simulink model "MagLev"  (R2015a)
settings: Solver=ode5  SolverMode=SingleTasking  StartTime=0.0  StopTime=5  FixedStep=1e-3  MaxStep=0.001  RelTol=1e-3  AbsTol=1e-5
PreLoadFcn:
  | Ts=1e-3;
libraries: vrlib x3
Description:
  | Magnetic Levitation Model
  | 
  | vrmaglev is an example showing the interaction between dynamic models in Simulink(R)
  | and virtual worlds. The Simulink model represents the HUMUSOFT(R) CE152 Magnetic Levitation
  | educational / presentation scale model. (http://www.humusoft.com/link/models)
  | 
  | The plant model is controlled by a PID controller with feed forward to cope with the nonlinearity
  | of the magnetic levitation system.
  | 
  | The position of the ball responds to the changing value of the setpoint. You can observe
  | this change not only in the Scope window, but also in a viewer window displaying
  | the virtual world. Note that the position of the ball represents the real dynamics of the system.
  | If you switch the VRML viewer to the Camera 3 viewpoint, you can observe and control the ball easier.
  | 
  | There are two possible methods of setting the ball position setpoint - using a Signal Generator
  | and visually by clicking at a desired position in the virtual reality scene.
  | 
  | In the virtual scene, a VRML sensor is defined. If you click in the space between the magnetic coil
  | and the bottom plate, VRML sensor is updated and its value is read into Simulink model using the
  | VR Source block.
settings Model: FPTRunName=Active  CovMetricSettings=d  CovSFcnEnable=off  ExtModeTrigDuration=5000  ExtModeTrigLevel=0.500000  Creator=The MathWorks Inc.  LastModifiedBy=Logan
settings DataIOCC: LimitDataPoints=off  SaveOutput=off  SaveTime=off  SignalLoggingName=logsOut
settings OptimizationCC: BlockReduction=off  BooleanDataType=off  OptimizeBlockIOStorage=off  BufferReuse=off  GlobalBufferReuse=off  ExpressionFolding=off  ExpressionDepthLimit=2147483647  LocalBlockOutputs=off  InitFltsAndDblsToZero=on
settings DebuggingCC: UnderspecifiedInitializationDetection=Classic  MergeDetectMultiDrivingBlocksExec=none  CheckExecutionContextPreStartOutputMsg=on  CheckExecutionContextRuntimeOutputMsg=on  SignalResolutionControl=TryResolveAllWithWarning  MultiTaskDSMMsg=warning  MultiTaskCondExecSysMsg=none  FcnCallInpInsideContextMsg=UseLocalSettings  StateNameClashWarn=warning
settings HardwareCC: TargetUnknown=on
settings ModelReferenceCC: UpdateModelReferenceTargets=IfOutOfDate
settings RTWCC: RetainRTWFile=on
settings GRTTargetCC: TargetFcnLib=ansi_tfl_tmw.mat  CombineOutputUpdateFcns=off  GRTInterface=on

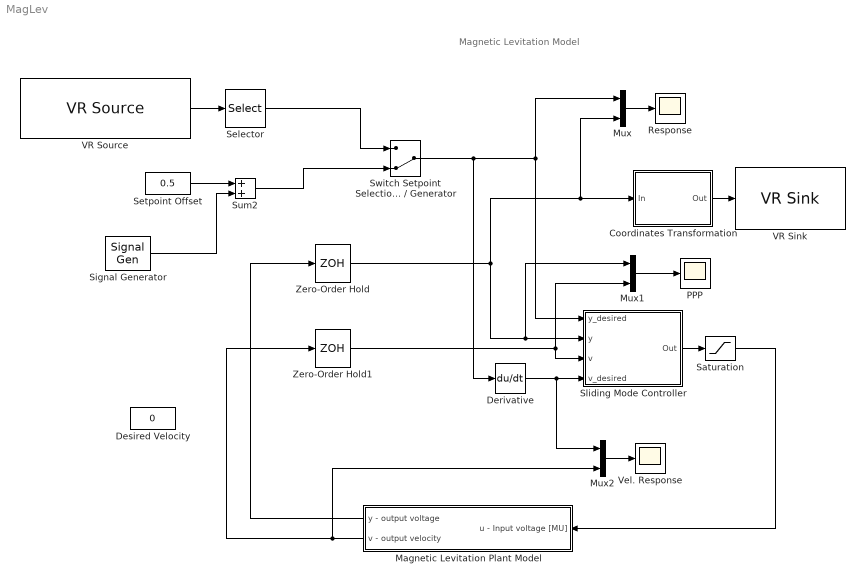
== system MagLev ==
  note: Magnetic Levitation Model
  Coordinates Transformation : Subsystem
  Derivative : Derivative
  Desired Velocity : Constant  Value=0
  Magnetic Levitation Plant Model : Subsystem
  Mux : Mux  Inputs=2
  Mux1 : Mux  Inputs=2
  Mux2 : Mux  Inputs=2
  PPP : Scope
      settings: TimeRange=5  YMin=0  YMax=1  SaveName=PhasePlane  MaxDataPoints=250  SampleInput=on  SampleTime=0.02
  Response : Scope
      settings: TimeRange=5  YMin=-0.0227122  YMax=1.027  SaveName=ResponseSMC  MaxDataPoints=250  SampleInput=on  SampleTime=0.02
  Saturation : Saturate  UpperLimit=1  LowerLimit=0  ZeroCross=off
  Selector : Selector  InputPortWidth=3  Indices=[2]
  Setpoint Offset : Constant  Value=0.5
  Signal Generator : SignalGenerator  Amplitude=0.25  Frequency=2  Units=rad/sec
  Sliding Mode Controller : Subsystem
  Sum2 : Sum  SaturateOnIntegerOverflow=on  InputSameDT=on  OutDataTypeStr=Inherit: Same as first input
  Switch Setpoint Selection Method Virtual Reality / Generator : ManualSwitch  CurrentSetting=0
  VR Sink : vrlib/VR Sink  InstantiateOnLoad=on  SampleTime=0.02  ViewEnable=on  RemoteChange=off  RemoteView=off  FieldsWritten=Ball.translation.3.1.1.double  WorldFileName=maglev.wrl  WorldDescription=VR Magnetic Levitation Model  AutoView=on  VideoDimensions=[]  AllowVariableSize=off
  VR Source : vrlib/VR Source  InstantiateOnLoad=on  SampleTime=0.1  ViewEnable=on  RemoteChange=off  RemoteView=off  FieldsRead=Grab_Sensor.translation_changed.3.1.1.double  WorldFileName=maglev.wrl  WorldDescription=VR Magnetic Levitation Model  AutoView=off  VideoDimensions=[]  AllowVariableSize=off
  Vel. Response : Scope
      settings: TimeRange=5  YMin=-0.0227122  YMax=1.027  DataFormat=Structure  MaxDataPoints=250  SampleInput=on  SampleTime=0.02
  Zero-Order Hold : ZeroOrderHold  SampleTime=Ts
  Zero-Order Hold1 : ZeroOrderHold  SampleTime=Ts
  wires:
  Zero-Order Hold/1 -> Coordinates Transformation/1(In), Mux/2, Mux1/1, Sliding Mode Controller/2(y)
  Switch Setpoint Selection Method Virtual Reality / Generator/1 -> Derivative/1, Sliding Mode Controller/1(y_desired), Mux/1
  Mux/1 -> Response/1
  Magnetic Levitation Plant Model/1(y - output voltage) -> Zero-Order Hold/1
  Coordinates Transformation/1(Out) -> VR Sink/1
  Saturation/1 -> Magnetic Levitation Plant Model/1(u - Input voltage [MU])
  Selector/1 -> Switch Setpoint Selection Method Virtual Reality / Generator/1
  VR Source/1 -> Selector/1
  Sliding Mode Controller/1(Out) -> Saturation/1
  Magnetic Levitation Plant Model/2(v - output velocity) -> Mux2/2, Zero-Order Hold1/1
  Zero-Order Hold1/1 -> Sliding Mode Controller/3(v), Mux1/2
  Mux1/1 -> PPP/1
  Signal Generator/1 -> Sum2/2
  Setpoint Offset/1 -> Sum2/1
  Sum2/1 -> Switch Setpoint Selection Method Virtual Reality / Generator/2
  Mux2/1 -> Vel. Response/1
  Derivative/1 -> Mux2/1, Sliding Mode Controller/4(v_desired)

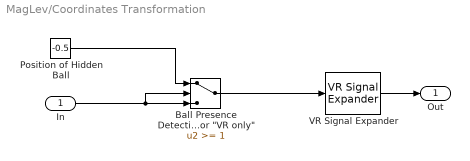
== system MagLev/Coordinates Transformation ==
  In : Inport
  "Ball Presence Detection Value > Threshold = Ball Not Present 1 for \"VR only\"" : Switch  Threshold=1  InputSameDT=on
  Position of Hidden Ball : Constant  Value=-0.5
  VR Signal Expander : vrlib/VR Signal Expander  outwidth=3  outidx=[2]
  Out : Outport
  wires:
  Position of Hidden Ball/1 -> "Ball Presence Detection Value > Threshold = Ball Not Present 1 for \"VR only\""/1
  In/1 -> "Ball Presence Detection Value > Threshold = Ball Not Present 1 for \"VR only\""/3, "Ball Presence Detection Value > Threshold = Ball Not Present 1 for \"VR only\""/2
  "Ball Presence Detection Value > Threshold = Ball Not Present 1 for \"VR only\""/1 -> VR Signal Expander/1
  VR Signal Expander/1 -> Out/1

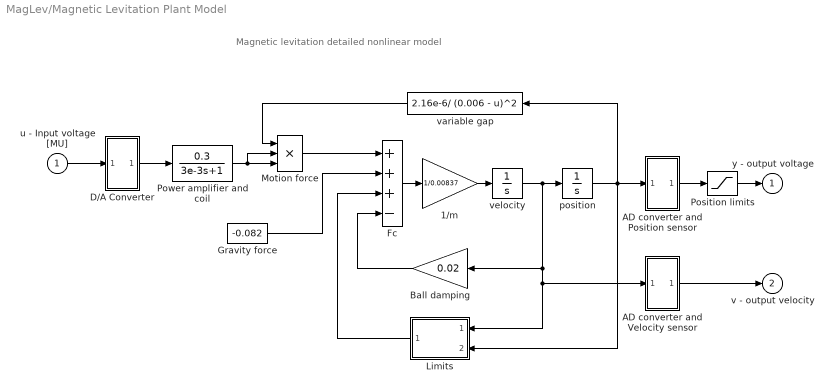
== system MagLev/Magnetic Levitation Plant Model ==
  note: Magnetic levitation
      | detailed nonlinear model
  u - Input voltage [MU] : Inport
  1/m : Gain  Gain=1/0.00837  SaturateOnIntegerOverflow=on  OutDataTypeStr=Inherit: Same as input  ParamDataTypeStr=Inherit: Same as input
  AD converter and Position sensor : Subsystem
      mask Display: disp('A/D')
  AD converter and Velocity sensor : Subsystem
      mask Display: disp('A/D')
  Ball damping : Gain  Gain=0.02  SaturateOnIntegerOverflow=on  OutDataTypeStr=Inherit: Same as input  ParamDataTypeStr=Inherit: Same as input
  D/A Converter : Subsystem
      mask Display: disp('D/A')
  Fc : Sum  Inputs=+++-  SaturateOnIntegerOverflow=on  InputSameDT=on  OutDataTypeStr=Inherit: Same as first input
  Gravity force : Constant  Value=-0.082
  Limits : Subsystem
      mask Display: disp('LIMIT')
  Motion force : Product  Inputs=3  SaturateOnIntegerOverflow=on  InputSameDT=on  OutDataTypeStr=Inherit: Same as first input
  Position limits : Saturate  UpperLimit=0.998  LowerLimit=0  ZeroCross=off
  Power amplifier and coil : TransferFcn  Numerator=[0.3]  Denominator=[3e-3 1]
  position : Integrator  LimitOutput=on  UpperSaturationLimit=0.005  LowerSaturationLimit=0  ZeroCross=off
  variable gap : Fcn  Expr=2.16e-6/ (0.006 - u)^2
  velocity : Integrator  UpperSaturationLimit=Inf  LowerSaturationLimit=-Inf  ZeroCross=off
  y - output voltage : Outport
  v - output velocity : Outport  Port=2
  wires:
  Ball damping/1 -> Fc/4
  variable gap/1 -> Motion force/1
  1/m/1 -> velocity/1
  Fc/1 -> 1/m/1
  Motion force/1 -> Fc/1
  Gravity force/1 -> Fc/2
  D/A Converter/1(out_1) -> Power amplifier and coil/1
  u - Input voltage [MU]/1 -> D/A Converter/1(in_1)
  AD converter and Position sensor/1(out_1) -> Position limits/1
  position/1 -> Limits/2(position), variable gap/1, AD converter and Position sensor/1(in_1)
  Limits/1(force) -> Fc/3
  Power amplifier and coil/1 -> Motion force/3, Motion force/2
  Position limits/1 -> y - output voltage/1
  AD converter and Velocity sensor/1(out_1) -> v - output velocity/1
  velocity/1 -> AD converter and Velocity sensor/1(in_1), Limits/1(velocity), Ball damping/1, position/1

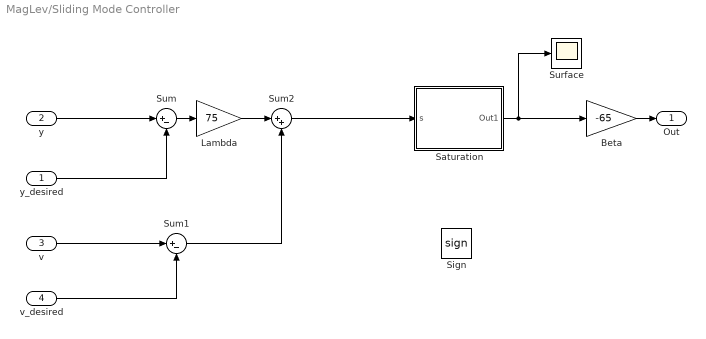
== system MagLev/Sliding Mode Controller ==
  y_desired : Inport
  y : Inport  Port=2
  v : Inport  Port=3
  v_desired : Inport  Port=4
  Beta : Gain  Gain=-65
  Lambda : Gain  Gain=75
  Saturation : Subsystem
  Sign : Signum
  Sum : Sum  Inputs=|+-
  Sum1 : Sum  Inputs=|+-
  Sum2 : Sum  Inputs=|++
  Surface : Scope
      settings: TimeRange=5  YMin=-3.15  YMax=-2.85  SaveName=ScopeData2  DataFormat=Structure  MaxDataPoints=250  SampleInput=on  SampleTime=0.02
  Out : Outport
  wires:
  v/1 -> Sum1/1
  v_desired/1 -> Sum1/2
  y/1 -> Sum/1
  y_desired/1 -> Sum/2
  Sum/1 -> Lambda/1
  Lambda/1 -> Sum2/1
  Sum1/1 -> Sum2/2
  Beta/1 -> Out/1
  Saturation/1(Out1) -> Surface/1, Beta/1
  Sum2/1 -> Saturation/1(s)

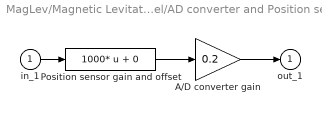
== system MagLev/Magnetic Levitation Plant Model/AD converter and Position sensor ==
  in_1 : Inport
  A/D converter gain : Gain  Gain=0.2  SaturateOnIntegerOverflow=on  OutDataTypeStr=Inherit: Same as input  ParamDataTypeStr=Inherit: Same as input
  Position sensor gain and offset : Fcn  Expr=1000* u + 0
  out_1 : Outport
  wires:
  in_1/1 -> Position sensor gain and offset/1
  Position sensor gain and offset/1 -> A/D converter gain/1
  A/D converter gain/1 -> out_1/1

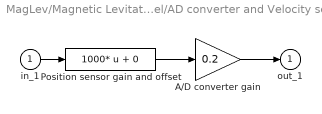
== system MagLev/Magnetic Levitation Plant Model/AD converter and Velocity sensor ==
  in_1 : Inport
  A/D converter gain : Gain  Gain=0.2  SaturateOnIntegerOverflow=on  OutDataTypeStr=Inherit: Same as input  ParamDataTypeStr=Inherit: Same as input
  Position sensor gain and offset : Fcn  Expr=1000* u + 0
  out_1 : Outport
  wires:
  in_1/1 -> Position sensor gain and offset/1
  Position sensor gain and offset/1 -> A/D converter gain/1
  A/D converter gain/1 -> out_1/1

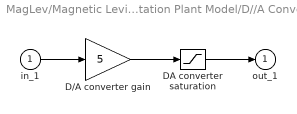
== system MagLev/Magnetic Levitation Plant Model/D//A Converter ==
  in_1 : Inport
  D/A converter gain : Gain  Gain=5  SaturateOnIntegerOverflow=on  OutDataTypeStr=Inherit: Same as input  ParamDataTypeStr=Inherit: Same as input
  DA converter saturation : Saturate  UpperLimit=5  LowerLimit=-5  ZeroCross=off
  out_1 : Outport
  wires:
  in_1/1 -> D/A converter gain/1
  DA converter saturation/1 -> out_1/1
  D/A converter gain/1 -> DA converter saturation/1

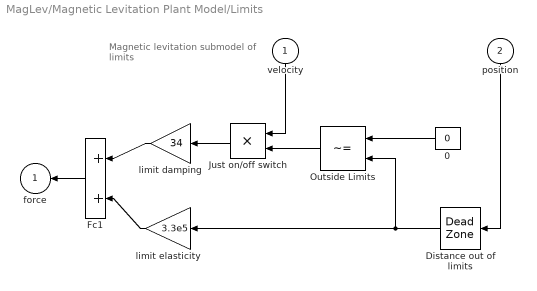
== system MagLev/Magnetic Levitation Plant Model/Limits ==
  note: Magnetic levitation
      | submodel of limits
  velocity : Inport
  position : Inport  Port=2
  0 : Constant  Value=0
  Distance out of limits : DeadZone  LowerValue=0  UpperValue=0.005  ZeroCross=off  SaturateOnIntegerOverflow=on
  Fc1 : Sum  SaturateOnIntegerOverflow=on  InputSameDT=on  OutDataTypeStr=Inherit: Same as first input
  "Just on/off switch " : Product  SaturateOnIntegerOverflow=on  InputSameDT=on  OutDataTypeStr=Inherit: Same as first input
  Outside Limits : RelationalOperator  Operator=~=  InputSameDT=on
  limit damping : Gain  Gain=34  SaturateOnIntegerOverflow=on  OutDataTypeStr=Inherit: Same as input  ParamDataTypeStr=Inherit: Same as input
  limit elasticity : Gain  Gain=3.3e5  SaturateOnIntegerOverflow=on  OutDataTypeStr=Inherit: Same as input  ParamDataTypeStr=Inherit: Same as input
  force : Outport
  wires:
  Distance out of limits/1 -> Outside Limits/2, limit elasticity/1
  limit damping/1 -> Fc1/1
  limit elasticity/1 -> Fc1/2
  Outside Limits/1 -> "Just on/off switch "/2
  0/1 -> Outside Limits/1
  "Just on/off switch "/1 -> limit damping/1
  velocity/1 -> "Just on/off switch "/1
  Fc1/1 -> force/1
  position/1 -> Distance out of limits/1

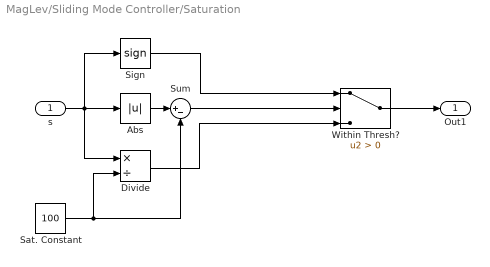
== system MagLev/Sliding Mode Controller/Saturation ==
  s : Inport
  Abs : Abs
  Divide : Product  Inputs=*/
  Sat. Constant : Constant  Value=100
  Sign : Signum
  Sum : Sum  Inputs=|+-
  Within Thresh? : Switch  Criteria=u2 > Threshold
  Out1 : Outport
  wires:
  s/1 -> Divide/1, Abs/1, Sign/1
  Within Thresh?/1 -> Out1/1
  Sign/1 -> Within Thresh?/1
  Divide/1 -> Within Thresh?/3
  Sat. Constant/1 -> Sum/2, Divide/2
  Abs/1 -> Sum/1
  Sum/1 -> Within Thresh?/2
